simulink model "KineMPC_22b"  (R2022b)
settings: Solver=ode8  StartTime=0.0  StopTime=8  FixedStep=Ts_plant  RelTol=1e-3
values from neighbouring files (symbols this model uses):
  Dm1 = 0.0    (= 0)    [SimParameters.m]    (also in param.mat)
  Dm2 = 0    [SimParameters.m]    (also in param.mat)
  Dm3 = 0    [SimParameters.m]    (also in param.mat)
  Jm1 = 8.61827e-4    (= 0.000861827)    [SimParameters.m]    (also in param.mat)
  Jm2 = 4.6370e-04    (= 0.0004637)    [SimParameters.m]    (also in param.mat)
  Jm3 = 2.4640e-04    (= 0.0002464)    [SimParameters.m]    (also in param.mat)
  Kpp1 = 2.0    (= 2)    [SimParameters.m]    (also in param.mat = 10)
  Kpp2 = 2.0    (= 2)    [SimParameters.m]    (also in param.mat = 10)
  Kpp3 = 2.0    (= 2)    [SimParameters.m]    (also in param.mat = 10)
  Kt1 = 4* 0.070504    (= 0.282016)    [SimParameters.m]    (also in param.mat)
  Kt2 = (0.07354) * (4)    (= 0.29416)    [SimParameters.m]    (also in param.mat)
  Kt3 = (0.0631765) * (4)    (= 0.252706)    [SimParameters.m]    (also in param.mat)
  Kvi1 = (w1*w1*Jm1)/Kt1    (= 7.6398768155)    [SimParameters.m]    (also in param.mat)
  Kvi2 = (w2*w2*Jm2)/Kt2    (= 3.94088251292)    [SimParameters.m]    (also in param.mat)
  Kvi3 = (w3*w3*Jm3)/Kt3    (= 2.43761525251)    [SimParameters.m]    (also in param.mat)
  Kvp1 = (Jm1*w1*zeta1)/Kt1    (= 0.15279753631)    [SimParameters.m]    (also in param.mat)
  Kvp2 = (Jm2*w2*zeta2)/Kt2    (= 0.0788176502584)    [SimParameters.m]    (also in param.mat)
  Kvp3 = (Jm3*w3*zeta3)/Kt3    (= 0.0487523050501)    [SimParameters.m]    (also in param.mat)
  Ts_control = 100e-6    (= 0.0001)    [SimParameters.m]    (also in param.mat)
settings Model: Creator=Juan  LastModifiedBy=user
settings DebuggingCC: UnderSpecifiedDimensionMsg=warning

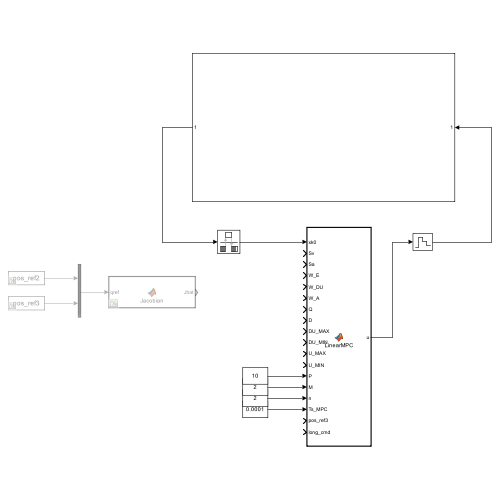
[thumbnail: Simulink's stored preview of the top-level diagram]
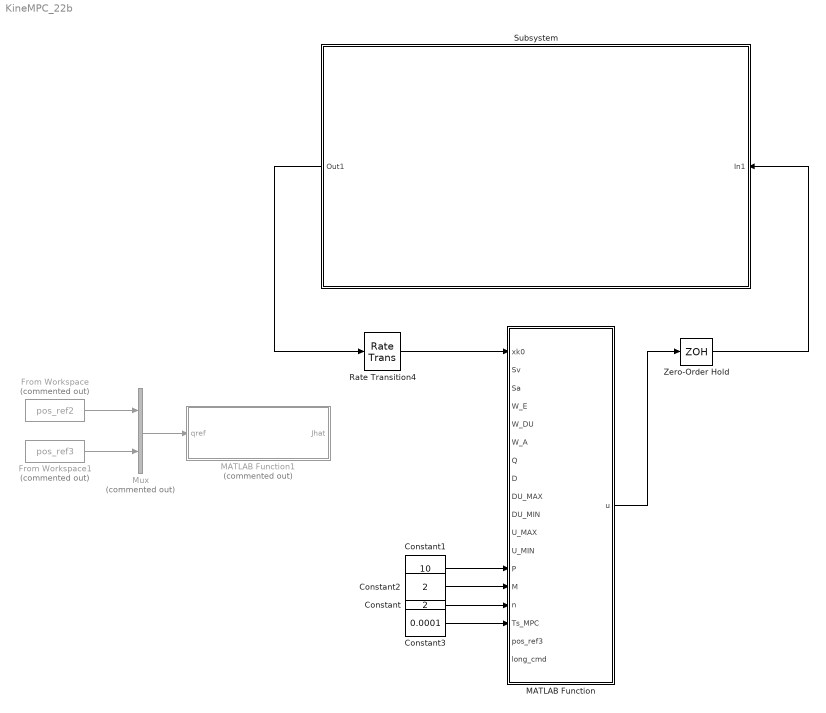
== system KineMPC_22b ==
  Constant : Constant  Value=2
  Constant1 : Constant  Value=10
  Constant2 : Constant  Value=2
  Constant3 : Constant  Value=0.0001
  From Workspace : FromWorkspace  Commented=on  VariableName=pos_ref2
  From Workspace1 : FromWorkspace  Commented=on  VariableName=pos_ref3
  MATLAB Function : MATLAB Function  TreatAsAtomicUnit=on
  MATLAB Function1 : MATLAB Function  Commented=on  TreatAsAtomicUnit=on
  Mux : Mux  Commented=on  Inputs=2
  Rate Transition4 : RateTransition  OutPortSampleTime=Ts_MPC
  Subsystem : Subsystem
  Zero-Order Hold : ZeroOrderHold  SampleTime=Ts_control
  wires:
  Rate Transition4/1 -> MATLAB Function/1(xk0)
  Mux/1 -> MATLAB Function1/1(qref)
  MATLAB Function/1(u) -> Zero-Order Hold/1
  Zero-Order Hold/1 -> Subsystem/1(In1)
  Subsystem/1(Out1) -> Rate Transition4/1
  From Workspace/1 -> Mux/1
  From Workspace1/1 -> Mux/2
  Constant/1 -> MATLAB Function/15(n)
  Constant1/1 -> MATLAB Function/13(P)
  Constant2/1 -> MATLAB Function/14(M)
  Constant3/1 -> MATLAB Function/16(Ts_MPC)

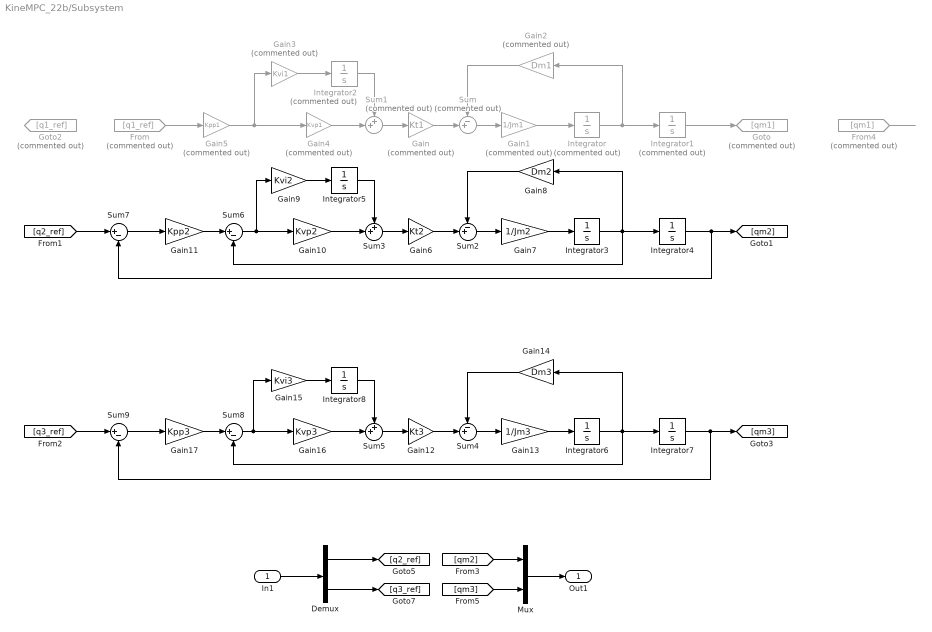
== system KineMPC_22b/Subsystem ==
  In1 : Inport
  Demux : Demux  Outputs=2
  From : From  Commented=on  GotoTag=q1_ref
  From4 : From  Commented=on  GotoTag=qm1
  Gain : Gain  Commented=on  Gain=Kt1
  Gain1 : Gain  Commented=on  Gain=1/Jm1
  Gain10 : Gain  Gain=Kvp2
  Gain11 : Gain  Gain=Kpp2
  Gain12 : Gain  Gain=Kt3
  Gain13 : Gain  Gain=1/Jm3
  Gain14 : Gain  Gain=Dm3
  Gain15 : Gain  Gain=Kvi3
  Gain16 : Gain  Gain=Kvp3
  Gain17 : Gain  Gain=Kpp3
  Gain2 : Gain  Commented=on  Gain=Dm1
  Gain3 : Gain  Commented=on  Gain=Kvi1
  Gain4 : Gain  Commented=on  Gain=Kvp1
  Gain5 : Gain  Commented=on  Gain=Kpp1
  Gain6 : Gain  Gain=Kt2
  Gain7 : Gain  Gain=1/Jm2
  Gain8 : Gain  Gain=Dm2
  Gain9 : Gain  Gain=Kvi2
  Goto : Goto  Commented=on  GotoTag=qm1
  Goto2 : Goto  Commented=on  GotoTag=q1_ref
  Integrator : Integrator  Commented=on
  Integrator1 : Integrator  Commented=on
  Integrator2 : Integrator  Commented=on
  Integrator{3..8} (6 alike) : Integrator
  Mux : Mux  Inputs=2
  Sum : Sum  Commented=on  Inputs=-+|
  Sum1 : Sum  Commented=on  Inputs=++|
  Sum2 : Sum  Inputs=-+|
  Sum3 : Sum  Inputs=++|
  Sum4 : Sum  Inputs=-+|
  Sum5 : Sum  Inputs=++|
  Sum{6..9} (4 alike) : Sum  Inputs=|+-
  Out1 : Outport
  wires:
  Gain1/1 -> Integrator/1
  Integrator/1 -> Gain2/1, Integrator1/1
  Integrator1/1 -> Goto/1
  Sum/1 -> Gain1/1
  In1/1 -> Demux/1
  Demux/1 -> [q2_ref]
  Demux/2 -> [q3_ref]
  Gain2/1 -> Sum/1
  Gain/1 -> Sum/2
  Sum1/1 -> Gain/1
  Gain3/1 -> Integrator2/1
  Integrator2/1 -> Sum1/1
  Gain4/1 -> Sum1/2
  Gain5/1 -> Gain3/1, Gain4/1
  From/1 -> Gain5/1
  [q2_ref] -> Sum7/1
  Gain10/1 -> Sum3/2
  Integrator5/1 -> Sum3/1
  Gain8/1 -> Sum2/1
  Gain9/1 -> Integrator5/1
  Gain6/1 -> Sum2/2
  Sum2/1 -> Gain7/1
  Integrator4/1 -> Sum7/2, [qm2]
  Gain7/1 -> Integrator3/1
  Integrator3/1 -> Sum6/2, Gain8/1, Integrator4/1
  Sum3/1 -> Gain6/1
  [q3_ref] -> Sum9/1
  Gain16/1 -> Sum5/2
  Integrator8/1 -> Sum5/1
  Gain14/1 -> Sum4/1
  Gain15/1 -> Integrator8/1
  Gain12/1 -> Sum4/2
  Sum4/1 -> Gain13/1
  Integrator7/1 -> [qm3], Sum9/2
  Gain13/1 -> Integrator6/1
  Integrator6/1 -> Sum8/2, Gain14/1, Integrator7/1
  Sum5/1 -> Gain12/1
  Mux/1 -> Out1/1
  [qm2] -> Mux/1
  [qm3] -> Mux/2
  From4/1 -> ?
  Sum7/1 -> Gain11/1
  Gain11/1 -> Sum6/1
  Sum6/1 -> Gain9/1, Gain10/1
  Sum9/1 -> Gain17/1
  Gain17/1 -> Sum8/1
  Sum8/1 -> Gain15/1, Gain16/1

== matlab function KineMPC_22b/MATLAB Function1 ==
  data: Jhat output; qref input
function Jhat = Jacobian(qref)
% q1,2,3はdegで与える
%clear variables;
%q1 = 0;
%q2 = 0;
%q3 = 0;
% q1 = 0;
q2 = qref(1);
q3 = qref(2);


% リンク長
% Lac = 0.2685;
% Lb  = 0.16;
% Ld  = 0.0880;
Le  = 0.56;
% Lf  = 0.088;
Lg  = 0.13;
Lh1 = 0.145;
Lh2 = 0.455;
Lii = 0.04;
Lj  = 0.2;
Lk  = 0.05;

% L1 = Lb;
L2 = Le;
L3 = Lg + Lii;
L4 = Lh1 + Lh2 + Lj + Lk;

% q1,2,3はdegで与える。ここでradに変換。
% theta1 = q1 / 180 * pi;
theta2 = q2 / 180 * pi;
theta3 = q3 / 180 * pi;
%theta3 = 0 / 180 * pi;

% 三角関数
S1 = sin(0);
C1 = cos(0);
S2 = sin(theta2);
C2 = cos(theta2);
S23 = sin(theta2 + theta3);
C23 = cos(theta2 + theta3);

% 各要素の偏微分
% dxdthe1 = -S1*(L1 + L2*S2 + L3*S23 + L4*C23);
dxdthe2 = C1*(L2*C2 + L3*C23 - L4*S23);
dxdthe3 = C1*(L3*C23 - L4*S23);
% dydthe1 = C1*(L1 + L2*S2 + L3*S23 + L4*C23);
dydthe2 = S1*(L2*C2 - L3*C23 - L4*S23);
dydthe3 = S1*(L3*C23 - L4*S23);
% dzdthe1 = 0;
dzdthe2 = -L2*S2 - L3*S23 - L4*C23;
dzdthe3 = -L3*S23 - L4*C23;

Jhat = [dxdthe2 dxdthe3;
        dzdthe2 dzdthe3];
end

== matlab function KineMPC_22b/MATLAB Function ==
  data: u output; xk0 input; pos_ref2 parameter; Sv input; Sa input; W_E input; W_DU input; W_A input; Q input; D input; DU_MAX input; DU_MIN input; U_MAX input; U_MIN input; P input; M input size=1; n input; Ts_MPC input; pos_ref3 input; long_cmd input
function u = LinearMPC(xk0, pos_ref2, Sv, Sa, W_E, W_DU, W_A, Q, D, DU_MAX, DU_MIN, U_MAX, U_MIN, P, M, n, Ts_MPC, pos_ref3, long_cmd)
%{
LinearMPC for Simulink

Solve the following quadratic program for every sample:

min  0.5*z'*H*z + f'*z
z
    s.t.  Dz<=b

where z = [Up | epsilon]' = [u{k} u{k+2} u{k+3} ... u{k+l-1} epsilon]'


***Required parameters (Detailed explanation given below):
For cost function: [H, R1, R2, R3]
For inequality constraints: [D, DU_MAX, DU_MIN, X_MAX, X_MIN, U_MAX, U_MIN, AAbar]
For both: [P, M, LT, L]
(P: Prediction horizon, L: Control horizon, LT: Number of constrained states, M: Input dimension) 
(Use LinearMPCPrecomputer function to compute)


***Input arguments:
-xk0: Last sample state vector X
-uk0: Last sample input vector u
-y_ref: Reference

***Output:
-Up: Computed optimal input vector over prediction horizon
-epsilon: Slack variable value
-x_predic: Predicted state vector over prediction horizon

NOTE: Some matrices need to be multiplied either with xk0 or uk0 to form
the whole quadratic program to be solved, so the precomputed required
parameters are given as below:
%}
% M = 2;
persistent k;
persistent uk0;
persistent duk0;
if isempty(k)
    k = 1;
end
if k > (long_cmd-P+1)
    k = long_cmd-P+1;
end
if isempty(uk0)
    uk0 = zeros(M,1);
end
if isempty(duk0)
    duk0 = zeros(M,1);
end
qref2 = zeros(P,1);
qref3 = zeros(P,1);
qref2(:,1) = pos_ref2(k:k+P-1,1);
qref3(:,1) = pos_ref3(k:k+P-1,1);

%Reference and previous value generation
% qref_P = repmat(qref,P,1);
qref_P = zeros(M*P,1);
Jhat = zeros(M,M,P);
% Jhat_P = kron(eye(P),Jhat);
for c= 1:P
    qref_P(2*(c-1)+1,1) = qref2(c);
    qref_P(2*(c-1)+2,1) = qref3(c);

    % q1,2,3はdegで与える
    q2 = qref2(c);
    q3 = qref3(c);
    
    % リンク長
    Le  = 0.56;
    Lg  = 0.13;
    Lh1 = 0.145;
    Lh2 = 0.455;
    Lii = 0.04;
    Lj  = 0.2;
    Lk  = 0.05;
    
    L2 = Le;
    L3 = Lg + Lii;
    L4 = Lh1 + Lh2 + Lj + Lk;
    
    % q1,2,3はdegで与える。ここでradに変換。
    theta2 = q2 / 180 * pi;
    theta3 = q3 / 180 * pi;
    
    % 三角関数
    S2 = sin(theta2);
    C2 = cos(theta2);
    S23 = sin(theta2 + theta3);
    C23 = cos(theta2 + theta3);
    
    % 各要素の偏微分
    % dxdthe1 = -S1*(L1 + L2*S2 + L3*S23 + L4*C23);
    dxdthe2 = (L2*C2 + L3*C23 - L4*S23);
    dxdthe3 = (L3*C23 - L4*S23);
    % dydthe1 = C1*(L1 + L2*S2 + L3*S23 + L4*C23);
    % dydthe2 = S1*(L2*C2 - L3*C23 - L4*S23);
    % dydthe3 = S1*(L3*C23 - L4*S23);
    % dzdthe1 = 0;
    dzdthe2 = -L2*S2 - L3*S23 - L4*C23;
    dzdthe3 = -L3*S23 - L4*C23;
    
    Jhat(:,:,c) = [dxdthe2 dxdthe3;
                   dzdthe2 dzdthe3];
end
Jhat_P = blkdiag(Jhat(:,:,1),Jhat(:,:,2),Jhat(:,:,3),Jhat(:,:,4),Jhat(:,:,5),Jhat(:,:,6),Jhat(:,:,7),Jhat(:,:,8),Jhat(:,:,9),Jhat(:,:,10));
v = zeros(M*P,1);
v(1:M,:) = -uk0;
v = v/Ts_MPC;
a = zeros(M*P,1);
a(1:M,:) = -uk0-duk0;
a(M+1:2*M,:) = uk0;
a = a/(Ts_MPC*Ts_MPC);

%Cost function 1\2 * H'*z*H + f'*z
%H is already precomputed
%z = [Up | epsilon]^T , where Up-> R(MP x MP), epsilon-> R(1x1)
H = 2*(Jhat_P'*W_E*Jhat_P + Q);
f = 2*(v'*W_DU*Sv + a'*W_A*Sa - qref_P'*Jhat_P'*W_E*Jhat_P)';

%Constraints
%   D*z<=b     (inequality constraints)
%D is already precomputed, b needs to be computed
%Inequalities: [D, DU_MAX, DU_MIN, U_MAX, U_MIN] needs to be precomputed

BMAX_Q = U_MAX;
BMIN_Q = U_MIN;
BMAX_DQ = DU_MAX - v;
BMIN_DQ = DU_MIN - v;
BMAX = [BMAX_DQ;
        BMAX_Q;
        ];    
    
BMIN = [BMIN_DQ;
        BMIN_Q;        
        ];

b = [BMAX;
    -BMIN];

%Solve quadratic program
%{
min  0.5*z'*H*z + f'*z
z
    s.t.  Dz<=b

where z = [Up | epsilon]' = [u{k} u{k+2} u{k+3} ... u{k+L-1} epsilon]'
%}
N = n*P;
opt = mpcInteriorPointOptions;
opt.IntegrityChecks = true;
x0 = zeros(N,1); %Cold start
Deq = zeros(0,N);
beq = zeros(0,1);
z = [1 1 1 1]';
% [z,exitflag] = mpcInteriorPointSolver(H,f,D,b,Deq,beq,x0,opt);
u = z(1:2,1);
uk0 = u;
k = k+1;

end
